simulink model "simulink_model"  (R2022b)
settings: Solver=FixedStepDiscrete  StartTime=0.0  StopTime=1  FixedStep=0.2  RelTol=1e-3
settings Model: Creator=ahmed  LastModifiedBy=ahmed
settings SolverCC: AlgebraicLoopSolver=TrustRegion
settings DataIOCC: ReturnWorkspaceOutputs=off
settings OptimizationCC: DefaultParameterBehavior=Inlined  UseDivisionForNetSlopeComputation=on  GainParamInheritBuiltInType=on  UseFloatMulNetSlope=on  InlineInvariantSignals=on  PassReuseOutputArgsAs=Individual arguments  ZeroExternalMemoryAtStartup=off  ZeroInternalMemoryAtStartup=off  NoFixptDivByZeroProtection=on  EfficientFloat2IntCast=on  LifeSpan=1  OptimizeBlockOrder=speed  DifferentSizesBufferReuse=on  EfficientTunableParamExpr=on
settings DebuggingCC: ParameterTunabilityLossMsg=error  UnconnectedInputMsg=warning  UnconnectedOutputMsg=warning  UnconnectedLineMsg=warning  SFMachineParentedDataDiag=warning  ArithmeticOperatorsInVariantConditions=warning
settings HardwareCC: ProdBitPerInt=16  ProdBitPerPointer=16  ProdBitPerSizeT=16  ProdBitPerPtrDiffT=16  ProdLargestAtomicFloat=None  ProdWordSize=8  ProdLongLongMode=on  ProdHWDeviceType=Atmel->AVR  TargetBitPerPointer=64  TargetBitPerSizeT=64  TargetBitPerPtrDiffT=64  TargetLongLongMode=on  TargetIntDivRoundTo=Zero  TargetEndianess=LittleEndian  TargetWordSize=64  TargetHWDeviceType=Generic->MATLAB Host Computer  ProdEqTarget=off
settings ModelReferenceCC: EnableRefExpFcnMdlSchedulingChecks=on
settings SFSimCC: SimUseLocalCustomCode=off  MATLABDynamicMemAlloc=off  CustomCodeUndefinedFunction=UseInterfaceOnly
settings RTWCC: Description=Embedded Coder  SystemTargetFile=ert.tlc  TemplateMakefile=ert_default_tmf  GenerateReport=on  RTWUseLocalCustomCode=off  IncludeHyperlinkInReport=on  LaunchReport=on  GenerateTraceInfo=on  GenerateTraceReport=on  GenerateTraceReportSl=on  GenerateTraceReportSf=on  GenerateTraceReportEml=on  GenerateCodeMetricsReport=on
settings CodeAppCC: ForceParamTrailComments=on  IgnoreCustomStorageClasses=off  OperatorAnnotations=on  SimulinkDataObjDesc=on  SFDataObjDesc=on  CustomSymbolStrGlobalVar=rt$N$M  CustomSymbolStrType=$N$M  CustomSymbolStrFcn=$N$M$F  CustomSymbolStrMacro=$N$M  InsertBlockDesc=on
settings ERTTargetCC: TargetLangStandard=C99 (ISO)  GenerateSampleERTMain=on  IncludeMdlTerminateFcn=off  CombineSignalStateStructs=on  SuppressErrorStatus=on  SupportAbsoluteTime=off  SupportComplex=off  InlinedParameterPlacement=NonHierarchical  ERTCustomFileTemplate=example_file_process.tlc  ERTFilePackagingFormat=CompactWithDataFile

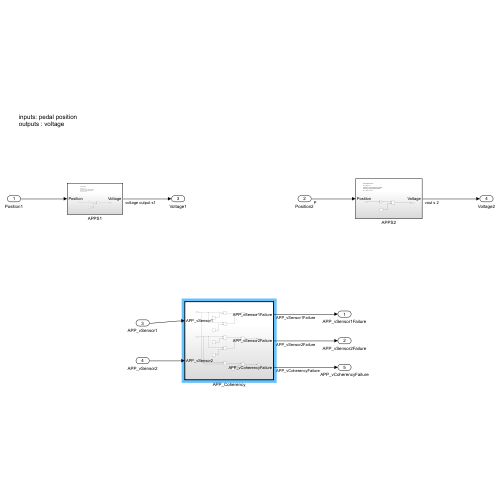
[thumbnail: Simulink's stored preview of the top-level diagram]
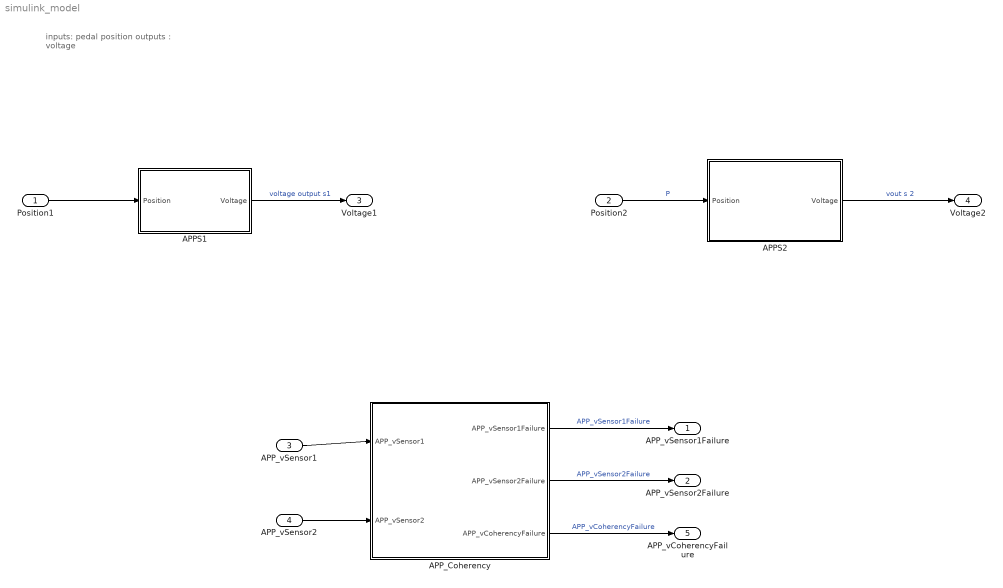
== system simulink_model ==
  note: inputs: pedal position
      | outputs : voltage
  Position1 : Inport
  Position2 : Inport  Port=2
  APP_vSensor1 : Inport  Port=3
  APP_vSensor2 : Inport  Port=4
  APPS1 : Subsystem
  APPS2 : Subsystem
  APP_Coherency : Subsystem  TreatAsAtomicUnit=on
  APP_vSensor1Failure : Outport  VectorParamsAs1DForOutWhenUnconnected=off
  APP_vSensor2Failure : Outport  Port=2  VectorParamsAs1DForOutWhenUnconnected=off
  Voltage1 : Outport  Port=3  VectorParamsAs1DForOutWhenUnconnected=off
  Voltage2 : Outport  Port=4  VectorParamsAs1DForOutWhenUnconnected=off
  APP_vCoherencyFailure : Outport  Port=5  VectorParamsAs1DForOutWhenUnconnected=off
  wires:
  APPS1/1(Voltage) -> Voltage1/1  "voltage output s1"
  APPS2/1(Voltage) -> Voltage2/1  "vout s 2"
  APP_vSensor1/1 -> APP_Coherency/1(APP_vSensor1)
  APP_vSensor2/1 -> APP_Coherency/2(APP_vSensor2)
  APP_Coherency/1(APP_vSensor1Failure) -> APP_vSensor1Failure/1  "APP_vSensor1Failure"
  APP_Coherency/2(APP_vSensor2Failure) -> APP_vSensor2Failure/1  "APP_vSensor2Failure"
  APP_Coherency/3(APP_vCoherencyFailure) -> APP_vCoherencyFailure/1  "APP_vCoherencyFailure"
  Position1/1 -> APPS1/1(Position)
  Position2/1 -> APPS2/1(Position)  "P"

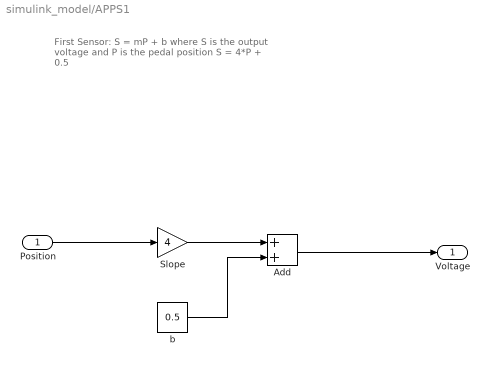
== system simulink_model/APPS1 ==
  note: First Sensor:
      | S = mP + b
      | where S is the output voltage
      | and P is the pedal position
      | S = 4*P + 0.5
  Position : Inport
  Add : Sum
  Slope : Gain  Gain=4
  "b " : Constant  Value=0.5
  Voltage : Outport  VectorParamsAs1DForOutWhenUnconnected=off
  wires:
  Slope/1 -> Add/1
  "b "/1 -> Add/2
  Add/1 -> Voltage/1
  Position/1 -> Slope/1

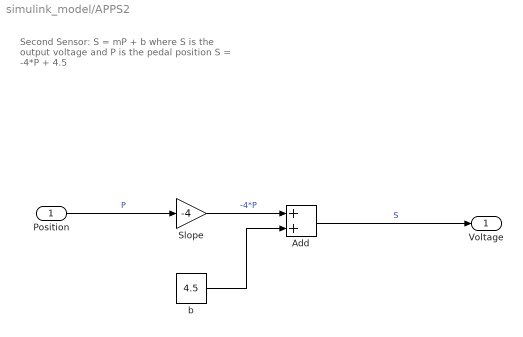
== system simulink_model/APPS2 ==
  note: Second Sensor:
      | S = mP + b
      | where S is the output voltage
      | and P is the pedal position
      | S = -4*P + 4.5
  Position : Inport
  Add : Sum
  Slope : Gain  Gain=-4
  "b " : Constant  Value=4.5
  Voltage : Outport  VectorParamsAs1DForOutWhenUnconnected=off
  wires:
  Slope/1 -> Add/1  "-4*P"
  Add/1 -> Voltage/1  "S"
  Position/1 -> Slope/1  "P"
  "b "/1 -> Add/2

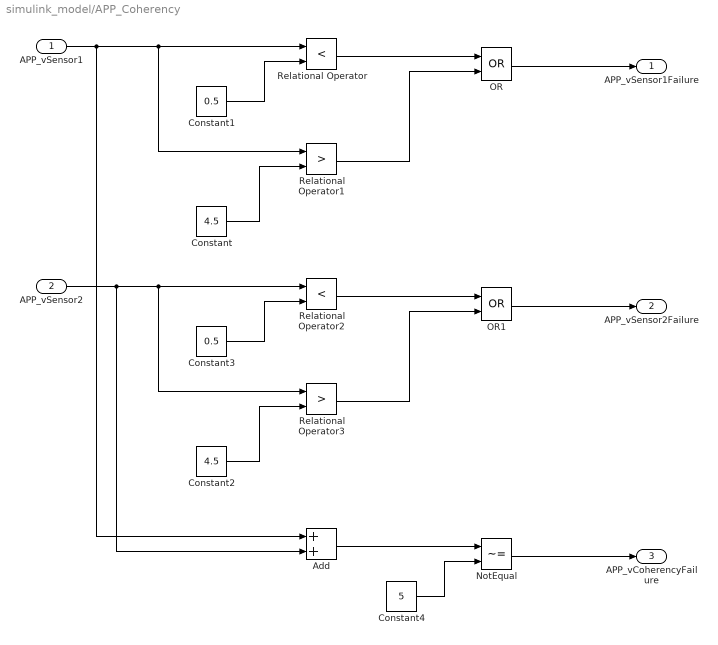
== system simulink_model/APP_Coherency ==
  APP_vSensor1 : Inport
  APP_vSensor2 : Inport  Port=2
  Add : Sum
  Constant : Constant  Value=4.5
  Constant1 : Constant  Value=0.5
  Constant2 : Constant  Value=4.5
  Constant3 : Constant  Value=0.5
  Constant4 : Constant  Value=5
  NotEqual : RelationalOperator  Operator=~=  OutDataTypeStr=boolean  RndMeth=Simplest  InputSameDT=off
  OR : Logic  Operator=OR  AllPortsSameDT=off  OutDataTypeStr=boolean
  OR1 : Logic  Operator=OR  AllPortsSameDT=off  OutDataTypeStr=boolean
  Relational Operator : RelationalOperator  Operator=<  OutDataTypeStr=boolean  RndMeth=Simplest  InputSameDT=off
  Relational Operator1 : RelationalOperator  Operator=>  OutDataTypeStr=boolean  RndMeth=Simplest  InputSameDT=off
  Relational Operator2 : RelationalOperator  Operator=<  OutDataTypeStr=boolean  RndMeth=Simplest  InputSameDT=off
  Relational Operator3 : RelationalOperator  Operator=>  OutDataTypeStr=boolean  RndMeth=Simplest  InputSameDT=off
  APP_vSensor1Failure : Outport  VectorParamsAs1DForOutWhenUnconnected=off
  APP_vSensor2Failure : Outport  Port=2  VectorParamsAs1DForOutWhenUnconnected=off
  APP_vCoherencyFailure : Outport  Port=3  VectorParamsAs1DForOutWhenUnconnected=off
  wires:
  APP_vSensor1/1 -> Add/1, Relational Operator/1, Relational Operator1/1
  Constant1/1 -> Relational Operator/2
  Relational Operator/1 -> OR/1
  Constant/1 -> Relational Operator1/2
  Relational Operator1/1 -> OR/2
  OR/1 -> APP_vSensor1Failure/1
  OR1/1 -> APP_vSensor2Failure/1
  APP_vSensor2/1 -> Add/2, Relational Operator2/1, Relational Operator3/1
  Constant3/1 -> Relational Operator2/2
  Constant2/1 -> Relational Operator3/2
  Relational Operator3/1 -> OR1/2
  Relational Operator2/1 -> OR1/1
  Add/1 -> NotEqual/1
  Constant4/1 -> NotEqual/2
  NotEqual/1 -> APP_vCoherencyFailure/1
